simulink model "SF007A_SysFricLrng"  (R2013b)
settings: Solver=FixedStepDiscrete  SolverMode=SingleTasking  StartTime=0.0  StopTime=1  FixedStep=0.002  RelTol=1e-3
PostLoadFcn:
  | , if any(exist('dsrtsu_mdlpostloadfcn', 'file') == [2, 3, 6]), try dsrtsu_mdlpostloadfcn('Execute', bdroot); catch fprintf('Error in PostLoadFcn (dsrtsu_mdlpostloadfcn) for model "%s":\n %s\n', bdroot, lasterr); end, end,
values from neighbouring files (symbols this model uses):
  ARCHGLBPRM_100MILLISEC_SEC_F32 = DataDict.Constant    [SF007A_SysFricLrng_DataDict.m]
  ARCHGLBPRM_10MILLISEC_SEC_F32 = DataDict.Constant    [SF007A_SysFricLrng_DataDict.m]
  ARCHGLBPRM_180OVERPI_ULS_F32 = DataDict.Constant    [SF007A_SysFricLrng_DataDict.m]
  CONV100MICROSECTOSEC_ULS_F32 = DataDict.Constant    [SF007A_SysFricLrng_DataDict.m]
  FLTINJ_SYSFRICLRNG_SYSFRICOFFS = DataDict.Constant    [SF007A_SysFricLrng_DataDict.m]
  FricLrngData = DataDict.NVM    [SF007A_SysFricLrng_DataDict.m]
  HWPTNUM_CNT_U08 = DataDict.Constant    [SF007A_SysFricLrng_DataDict.m]
  HWPTNUMSUB1_CNT_U08 = DataDict.Constant    [SF007A_SysFricLrng_DataDict.m]
  HWVELDECDIR_ULS_U08 = DataDict.Constant    [SF007A_SysFricLrng_DataDict.m]
  HWVELINCDIR_ULS_U08 = DataDict.Constant    [SF007A_SysFricLrng_DataDict.m]
  IDXCALCNSCAGFAC_ULS_U08 = DataDict.Constant    [SF007A_SysFricLrng_DataDict.m]
  IDXSELN1_ULS_U08 = DataDict.Constant    [SF007A_SysFricLrng_DataDict.m]
  IDXSELN2_ULS_U08 = DataDict.Constant    [SF007A_SysFricLrng_DataDict.m]
  IDXSELN3_ULS_U08 = DataDict.Constant    [SF007A_SysFricLrng_DataDict.m]
  LRNGENASCAFAC_MILLISEC_U32 = DataDict.Constant    [SF007A_SysFricLrng_DataDict.m]
  SCAGFACQUARTER_CNT_F32 = DataDict.Constant    [SF007A_SysFricLrng_DataDict.m]
  SCAGFACTEN_CNT_U16 = DataDict.Constant    [SF007A_SysFricLrng_DataDict.m]
  SCAGFACVEHLATA_MTRPERSECSQD_F32 = DataDict.Constant    [SF007A_SysFricLrng_DataDict.m]
  SECIDXSELN_ULS_U08 = DataDict.Constant    [SF007A_SysFricLrng_DataDict.m]
  SysFricLrngBasLineEolFric = DataDict.Calibration    [SF007A_SysFricLrng_DataDict.m]
  SysFricLrngBasLineFric = DataDict.Calibration    [SF007A_SysFricLrng_DataDict.m]
  SysFricLrngBasLineHys = DataDict.Calibration    [SF007A_SysFricLrng_DataDict.m]
  SysFricLrngBasLineRngCntr = DataDict.Calibration    [SF007A_SysFricLrng_DataDict.m]
  SysFricLrngEolFricDifScagFac = DataDict.Calibration    [SF007A_SysFricLrng_DataDict.m]
  SysFricLrngFricChgWght = DataDict.Calibration    [SF007A_SysFricLrng_DataDict.m]
  SysFricLrngFricDiagcThd = DataDict.Calibration    [SF007A_SysFricLrng_DataDict.m]
  SysFricLrngFricDiagcTiThd = DataDict.Calibration    [SF007A_SysFricLrng_DataDict.m]
  SysFricLrngFricHysHwAgPt = DataDict.Calibration    [SF007A_SysFricLrng_DataDict.m]
  SysFricLrngGain = DataDict.Calibration    [SF007A_SysFricLrng_DataDict.m]
  SysFricLrngHwPosnAuthyThd = DataDict.Calibration    [SF007A_SysFricLrng_DataDict.m]
  SysFricLrngHwVelConstrLim = DataDict.Calibration    [SF007A_SysFricLrng_DataDict.m]
  SysFricLrngHwVelHiLim = DataDict.Calibration    [SF007A_SysFricLrng_DataDict.m]
  SysFricLrngHwVelLoLim = DataDict.Calibration    [SF007A_SysFricLrng_DataDict.m]
  SysFricLrngIgnCycFricChgLim = DataDict.Calibration    [SF007A_SysFricLrng_DataDict.m]
  SysFricLrngLatAHiLim = DataDict.Calibration    [SF007A_SysFricLrng_DataDict.m]
  SysFricLrngLatALoLim = DataDict.Calibration    [SF007A_SysFricLrng_DataDict.m]
  SysFricLrngMaskVehSpd = DataDict.Calibration    [SF007A_SysFricLrng_DataDict.m]
  SysFricLrngRngCntrThd = DataDict.Calibration    [SF007A_SysFricLrng_DataDict.m]
  SysFricLrngThd = DataDict.Calibration    [SF007A_SysFricLrng_DataDict.m]
  SysFricLrngTHiLim = DataDict.Calibration    [SF007A_SysFricLrng_DataDict.m]
  SysFricLrngTLoLim = DataDict.Calibration    [SF007A_SysFricLrng_DataDict.m]
  SysFricLrngVehSpd = DataDict.Calibration    [SF007A_SysFricLrng_DataDict.m]
  SYSFRICOFFSLIM_HWNWTMTR_F32 = DataDict.Constant    [SF007A_SysFricLrng_DataDict.m]
  VEHSPDPTNUM1_ULS_U08 = DataDict.Constant    [SF007A_SysFricLrng_DataDict.m]
  VEHSPDPTNUM2_ULS_U08 = DataDict.Constant    [SF007A_SysFricLrng_DataDict.m]
undefined symbols (not defined in the file or in its folder): NtcNr1, NtcSts1, SysFricLrngOperMod1
libraries: Fil x19, simulink x17, NxtrLim x10, NxtrAbslt x3, NxtrNvM x2, FixdToFloat x2, FloatToFixd x1, LnrIntrpn x1
(part 1 of 7)
settings Model: DSRTSU_INTERNAL_RTI_VER=370  DSRTSU_INTERNAL_RTI_TYPE=rti1401  Creator=fzv52m  LastModifiedBy=VZBTJX
settings Model: ModifiedHistory=|
  | Ver 004 Removed ignition latching of Friction Detection NTC to match software.
  | Limiting of P steps to one per ignition is being done with latching NTC allowing for the change
settings SolverCC: AutoInsertRateTranBlk=on  InsertRTBMode=Always
settings DataIOCC: LimitDataPoints=off  SaveFormat=Structure  ReturnWorkspaceOutputs=on
settings OptimizationCC: BlockReduction=off  InlineParams=on  ZeroExternalMemoryAtStartup=off  ZeroInternalMemoryAtStartup=off  OptimizeModelRefInitCode=on  LifeSpan=1
settings DebuggingCC: SignalInfNanChecking=error  SignalRangeChecking=warning  UnderspecifiedInitializationDetection=Simplified  SolverPrmCheckMsg=error  InheritedTsInSrcMsg=error  DiscreteInheritContinuousMsg=error  SingleTaskRateTransMsg=error  TasksWithSamePriorityMsg=error  SigSpecEnsureSampleTimeMsg=error  CheckMatrixSingularityMsg=error  ParameterUnderflowMsg=error  ParameterPrecisionLossMsg=error  ParameterTunabilityLossMsg=error  FixptConstUnderflowMsg=warning  FixptConstOverflowMsg=warning  VectorMatrixConversionMsg=error  SignalLabelMismatchMsg=error  UnconnectedInputMsg=error  UnconnectedOutputMsg=error  UnconnectedLineMsg=error  SFcnCompatibilityMsg=error  UniqueDataStoreMsg=warning  BusObjectLabelMismatch=error  RootOutportRequireBusObject=error  AssertControl=DisableAll  ModelReferenceIOMsg=error  ModelReferenceVersionMismatchMessage=warning  ModelReferenceIOMismatchMessage=error  ModelReferenceCSMismatchMessage=warning  ModelReferenceDataLoggingMessage=error  StateNameClashWarn=warning  StrictBusMsg=ErrorOnBusTreatedAsVector  NonBusSignalsTreatedAsBus=error  SFUnexpectedBacktrackingDiag=error  SFInvalidInputDataAccessInChartInitDiag=error  SFNoUnconditionalDefaultTransitionDiag=error  SFTransitionOutsideNaturalParentDiag=error  SFUnconditionalTransitionShadowingDiag=error  SFUndirectedBroadcastEventsDiag=error
settings ModelReferenceCC: ModelReferenceNumInstancesAllowed=Single
settings SFSimCC: SimGenImportedTypeDefs=on
settings RTWCC: SystemTargetFile=autosar.tlc  GenCodeOnly=on  TemplateMakefile=ert_default_tmf  Description=AUTOSAR  GenerateReport=on  ProcessScript=autosar_make_rtw_hook  LaunchReport=on
settings CodeAppCC: GenerateComments=off  IgnoreCustomStorageClasses=off  CustomSymbolStrType=$N$R$M  CustomSymbolStrBlkIO=$N$M  SimulinkBlockComments=off
settings STFCustomTargetCC: ParMdlRefBuildCompliant=on  CompOptLevelCompliant=on  IncludeMdlTerminateFcn=off  CombineOutputUpdateFcns=on  SuppressErrorStatus=on  ERTFirstTimeCompliant=on  ERTCustomFileBanners=on  SupportNonFinite=off  SupportComplex=off  SupportContinuousTime=off  SupportNonInlinedSFcns=off  MATLABClassNameForMDSCustomization=Simulink.SoftwareTarget.ERTCustomization  AutosarCompliant=on  GRTInterface=off  SystemTargetFile=autosar.tlc
settings ERTTargetCC: CodeReplacementLibrary=ANSI_C  ConcurrentExecutionCompliant=off  IncludeMdlTerminateFcn=off  SuppressErrorStatus=on  SupportNonFinite=off  SupportComplex=off  ModelStepFunctionPrototypeControlCompliant=off  CPPClassGenCompliant=off  AutosarCompliant=on  InlinedParameterPlacement=NonHierarchical  ERTCustomFileTemplate=example_file_process.tlc  EnableUserReplacementTypes=on

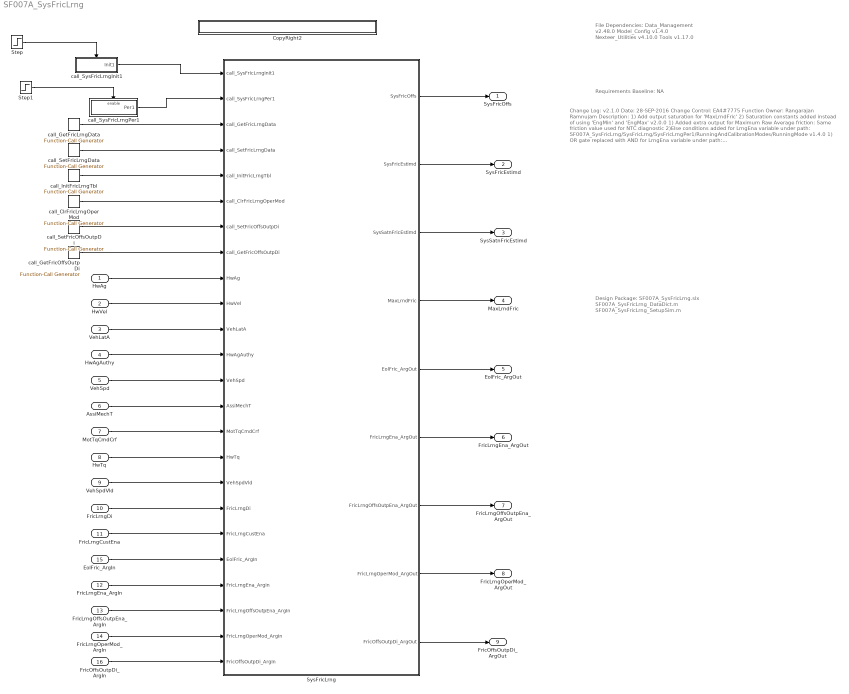
== system SF007A_SysFricLrng ==
  note: Requirements Baseline: NA
  note: File Dependencies:
      |
      | Data_Management v2.48.0
      | Model_Config v1.4.0
      | Nexteer_Utilities v4.10.0
      | Tools v1.17.0
  note: Change Log:
      |
      | v2.1.0
      | Date: 28-SEP-2016
      | Change Control: EA4#7775
      | Function Owner:  Rangarajan Ramnujam
      | Description:
      | 1) Add output saturation for 'MaxLrndFric'
      | 2) Saturation constants added instead of using 'EngMin' and 'EngMax'
      |
      | v2.0.0
      | 1) Added extra output for Maximum Raw Average friction: Same friction value used for NTC diagnostic
      | 2)Else conditions added for LrngEna variable under path:
      | SF007A_SysFricLrng/SysFricLrng/SysFricLrngPer1/RunningAndCalibrationModes/RunningMode
      |
      | v1.4.0
      | 1) OR gate replaced with AND for LrngEna variable under path:
      | SF007A_SysFricLrng/SysFricLrng/SysFricLrngPer1/RunningAndCalibrationModes
      | 2) Logic updated under path
      | SF007A_SysFricLrng/SysFricLrng/SysFricLrngPer1/RunningAndCalibrationModes/Running Mode
      | 3) Eng min to -127 and Eng max to 254 updated for PIM 'FilAvrgFric' in Data Dict
      | 4) Logic for Indices calculation updated under below path. This change needed only in model as
      |     model uses one based Index logic. No code change required for this.
      |     SF007A_SysFricLrng/SysFricLrng/SysFricLrngPer1/RunningAndCalibrationModes/FricLearning/Indices Calculation
      | - Changes are highlighted in red. Code change needed for above mentioned changes 1, 2, and 4.
      |
      | v1.3.1
      | Date: 18-JULY-2016
      | Change Control: EA4#6450
      | DRW:  Hari Prasad(KPIT)
      | Description:
      | - Anomaly EA4#6361 Fixing for Gate variable look up table indexing.
      |   Removed 'Gate_Cnt_T_u08' temporary data store memory block.
      |   Logic related to it has been updated.
      | - Changes are highlighted in red. No code change needed.
      |
      | v1.3.0
      | Date: 07-APR-2016
      | Change Control #4835:
      | DRW:  Muragesh Asundi
      | Description:
      | - List of issues fixed are available under
      |   Doc/SF007_FDD_Issues.xlsx/Issues in V1.2.0
      | - In below path, Changed Gate from PIM to port inside subsystem
      |  as PIM wholds extra increment inside while loop
      |   SF007A_SysFricLrng/SysFricLrng/SysFricLrngPer1/RunningAndCalibrationModes/
      |   FricLearning/Range Counter Manager/Range Counter Control
      |
      | v1.2.0
      | Date: 30-Mar-2016
      | Change Control #4835:
      | DR W:  Muragesh Asundi
      | Description:
      | - List of issues fixed are available under
      |   Doc/SF007_FDD_Issues.xlsx/Issues in V1.1.0
      | - 'SetFricLrngOperMod' renamed to 'SetFricLrngData'
      | - 'SetEolFric' removed and merged with 'SetFricLrngData'
      | - Following PIMs have been removed from model and DD
      | 'HwAgPrev', 'HwVelPrev', 'ColTq'
      | - Monotony of callibration table 'SysFricLrngFricHysHwAgPt'
      | changed to 'Strictly_Increasing'
      | - Init value of PIM 'TotCntr' changed to 1
      |
      | v1.1.0
      | Date: 25-Mar-2016
      | Change Control #4835:
      | DRW:  Hari Prasad
      | Description:
      | - List of issues fixed are available under
      |   Doc/SF007_FDD_Issues.xlsx
      | - Changes are highlighed in red color
      |
      | v1.0.0
      | Date: 11-Mar-2016
      | Change Control #2719:
      | DRW:  Hari Prasad, Muragesh Asundi
      | Description:
      | - Initial Release of EA4 from EA3 V008
  note: Design Package:
      |
      | SF007A_SysFricLrng.slx
      | SF007A_SysFricLrng_DataDict.m
      | SF007A_SysFricLrng_SetupSim.m
  HwAg : Inport
  HwVel : Inport  Port=2
  VehLatA : Inport  Port=3
  HwAgAuthy : Inport  Port=4
  VehSpd : Inport  Port=5
  AssiMechT : Inport  Port=6
  MotTqCmdCrf : Inport  Port=7
  HwTq : Inport  Port=8
  VehSpdVld : Inport  Port=9
  FricLrngDi : Inport  Port=10
  FricLrngCustEna : Inport  Port=11
  FricLrngEna_ArgIn : Inport  Port=12
  FricLrngOffsOutpEna_ArgIn : Inport  Port=13
  FricLrngOperMod_ArgIn : Inport  Port=14
  EolFric_ArgIn : Inport  Port=15
  FricOffsOutpDi_ArgIn : Inport  Port=16
  CopyRight2 : Subsystem  Description=|  mask(Copyright Information){none=on}
      | Copyright info block.                                               
      |                                                                     
      | Place copyright information at the top of every subsystem in design.
      mask prompts: none "No parameters"
      mask help: Place copyright information at the top of every subsystem in design.
      mask Display:
      | NxtrConf = 'Nexteer Confidential';
      | 
      | sys = bdroot; %handle for the current model ("system")
      | first = get_param(sys,'Created');
      | first = first(end-3:end);  %year is last four digits
      | 
      | last = get_param(sys,'LastModifiedDate');
      | if isempty(last)
      |     last = datestr(now,'yyyy');
      | else
      |     last = last(end-3:end);
      | end
      | 
      | if strcmp(first,last)
      |     fprintf('%s -- Copyright %s Nexteer',NxtrConf,first)
      | else
      |     fprintf('%s -- %s%s- %s Nexteer',NxtrConf,char(169),first,last)
      | end
  Step : Step  Time=.001  Before=1  After=0  SampleTime=0
  Step1 : Step  Time=.001  SampleTime=0
  SysFricLrng : Subsystem
  call_ClrFricLrngOperMod : simulink/Ports & Subsystems/Function-Call Generator  sample_time=0.010  numberOfIterations=1
  call_GetFricLrngData : simulink/Ports & Subsystems/Function-Call Generator  sample_time=0.010  numberOfIterations=1
  call_GetFricOffsOutpDi : simulink/Ports & Subsystems/Function-Call Generator  sample_time=0.010  numberOfIterations=1
  call_InitFricLrngTbl : simulink/Ports & Subsystems/Function-Call Generator  sample_time=0.010  numberOfIterations=1
  call_SetFricLrngData : simulink/Ports & Subsystems/Function-Call Generator  sample_time=0.010  numberOfIterations=1
  call_SetFricOffsOutpDi : simulink/Ports & Subsystems/Function-Call Generator  sample_time=0.010  numberOfIterations=1
  call_SysFricLrngInit1 : Subsystem  TreatAsAtomicUnit=on
  call_SysFricLrngPer1 : Subsystem  TreatAsAtomicUnit=on
  SysFricOffs : Outport
  SysFricEstimd : Outport  Port=2
  SysSatnFricEstimd : Outport  Port=3
  MaxLrndFric : Outport  Port=4
  EolFric_ArgOut : Outport  Port=5
  FricLrngEna_ArgOut : Outport  Port=6
  FricLrngOffsOutpEna_ArgOut : Outport  Port=7
  FricLrngOperMod_ArgOut : Outport  Port=8
  FricOffsOutpDi_ArgOut : Outport  Port=9
  wires:
  MotTqCmdCrf/1 -> SysFricLrng/15(MotTqCmdCrf)
  FricLrngDi/1 -> SysFricLrng/18(FricLrngDi)
  HwVel/1 -> SysFricLrng/10(HwVel)
  HwAg/1 -> SysFricLrng/9(HwAg)
  HwTq/1 -> SysFricLrng/16(HwTq)
  VehSpdVld/1 -> SysFricLrng/17(VehSpdVld)
  call_GetFricLrngData/1 -> SysFricLrng/3(call_GetFricLrngData)
  HwAgAuthy/1 -> SysFricLrng/12(HwAgAuthy)
  AssiMechT/1 -> SysFricLrng/14(AssiMechT)
  VehLatA/1 -> SysFricLrng/11(VehLatA)
  VehSpd/1 -> SysFricLrng/13(VehSpd)
  SysFricLrng/1(SysFricOffs) -> SysFricOffs/1
  SysFricLrng/3(SysSatnFricEstimd) -> SysSatnFricEstimd/1
  SysFricLrng/2(SysFricEstimd) -> SysFricEstimd/1
  FricLrngCustEna/1 -> SysFricLrng/19(FricLrngCustEna)
  call_SetFricLrngData/1 -> SysFricLrng/4(call_SetFricLrngData)
  call_InitFricLrngTbl/1 -> SysFricLrng/5(call_InitFricLrngTbl)
  call_SetFricOffsOutpDi/1 -> SysFricLrng/7(call_SetFricOffsOutpDi)
  call_GetFricOffsOutpDi/1 -> SysFricLrng/8(call_GetFricOffsOutpDi)
  call_ClrFricLrngOperMod/1 -> SysFricLrng/6(call_ClrFricLrngOperMod)
  SysFricLrng/6(FricLrngEna_ArgOut) -> FricLrngEna_ArgOut/1
  SysFricLrng/8(FricLrngOperMod_ArgOut) -> FricLrngOperMod_ArgOut/1
  SysFricLrng/7(FricLrngOffsOutpEna_ArgOut) -> FricLrngOffsOutpEna_ArgOut/1
  SysFricLrng/9(FricOffsOutpDi_ArgOut) -> FricOffsOutpDi_ArgOut/1
  SysFricLrng/5(EolFric_ArgOut) -> EolFric_ArgOut/1
  FricLrngEna_ArgIn/1 -> SysFricLrng/21(FricLrngEna_ArgIn)
  FricLrngOffsOutpEna_ArgIn/1 -> SysFricLrng/22(FricLrngOffsOutpEna_ArgIn)
  FricLrngOperMod_ArgIn/1 -> SysFricLrng/23(FricLrngOperMod_ArgIn)
  EolFric_ArgIn/1 -> SysFricLrng/20(EolFric_ArgIn)
  FricOffsOutpDi_ArgIn/1 -> SysFricLrng/24(FricOffsOutpDi_ArgIn)
  call_SysFricLrngInit1/1(Init1) -> SysFricLrng/1(call_SysFricLrngInit1)
  Step/1 -> call_SysFricLrngInit1/Enable
  call_SysFricLrngPer1/1(Per1) -> SysFricLrng/2(call_SysFricLrngPer1)
  Step1/1 -> call_SysFricLrngPer1/Enable
  SysFricLrng/4(MaxLrndFric) -> MaxLrndFric/1

== system SF007A_SysFricLrng/CopyRight2 ==

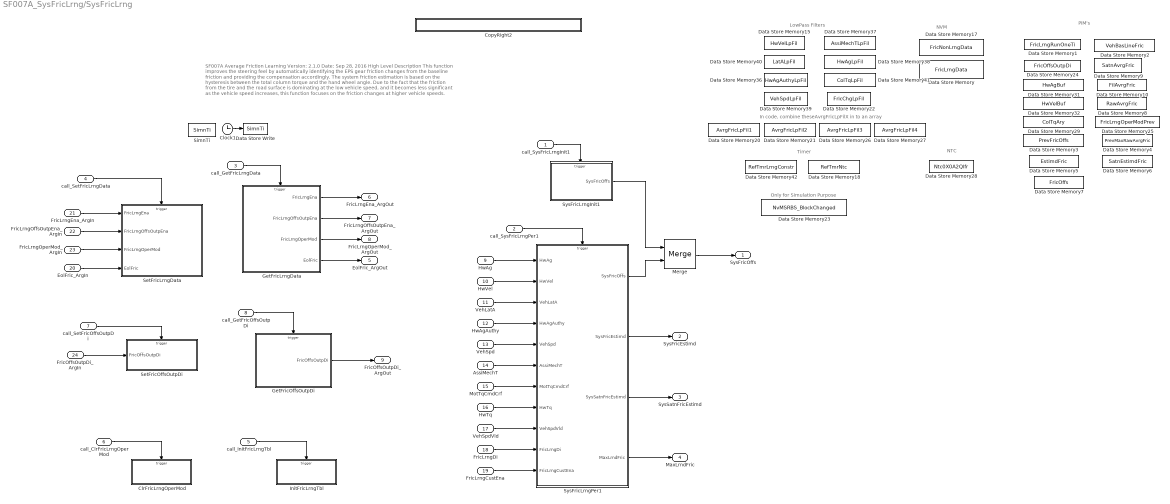
== system SF007A_SysFricLrng/SysFricLrng ==
  note: In code, combine theseAvrgFricLpFilX in to an array
  note: Only for Simulation Purpose
  note: PIM's
  note: Timer
  note: LowPass Filters
  note: NVM
  note: SF007A  Average Friction Learning
      | Version: 2.1.0          																															 					Date: Sep 28,  2016
      |
      | High Level Description
      |
      | This function improves the steering feel by automatically identifying the EPS gear friction changes from the baseline friction and providing the compensation accordingly. The system friction estimation
      |  is based on the hysteresis between the total column torque and the hand wheel angle. Due to the fact that the friction from the tire and the road surface is dominating at the low vehicle speed,  and it
      | becomes less significant as the vehicle speed increases, this function focuses on the friction changes at higher vehicle speeds.
  note: NTC
  call_SysFricLrngInit1 : Inport
  call_SysFricLrngPer1 : Inport  Port=2
  call_GetFricLrngData : Inport  Port=3
  call_SetFricLrngData : Inport  Port=4
  call_InitFricLrngTbl : Inport  Port=5
  call_ClrFricLrngOperMod : Inport  Port=6
  call_SetFricOffsOutpDi : Inport  Port=7
  call_GetFricOffsOutpDi : Inport  Port=8
  HwAg : Inport  Port=9
  HwVel : Inport  Port=10
  VehLatA : Inport  Port=11
  HwAgAuthy : Inport  Port=12
  VehSpd : Inport  Port=13
  AssiMechT : Inport  Port=14
  MotTqCmdCrf : Inport  Port=15
  HwTq : Inport  Port=16
  VehSpdVld : Inport  Port=17
  FricLrngDi : Inport  Port=18
  FricLrngCustEna : Inport  Port=19
  EolFric_ArgIn : Inport  Port=20
  FricLrngEna_ArgIn : Inport  Port=21
  FricLrngOffsOutpEna_ArgIn : Inport  Port=22
  FricLrngOperMod_ArgIn : Inport  Port=23
  FricOffsOutpDi_ArgIn : Inport  Port=24
  Clock1 : Clock
  ClrFricLrngOperMod : Subsystem
  CopyRight2 : Subsystem  Description=|  mask(Copyright Information){none=on}
      | Copyright info block.                                               
      |                                                                     
      | Place copyright information at the top of every subsystem in design.
      mask prompts: none "No parameters"
      mask help: Place copyright information at the top of every subsystem in design.
      mask Display:
      | NxtrConf = 'Nexteer Confidential';
      | 
      | sys = bdroot; %handle for the current model ("system")
      | first = get_param(sys,'Created');
      | if(isempty(first))
      |     first = datestr(now,'yyyy');
      | else
      |     first = first(end-3:end);  %year is last four digits
      | end
      | 
      | last = get_param(sys,'LastModifiedDate');
      | if isempty(last)
      |     last = datestr(now,'yyyy');
      | else
      |     last = last(end-3:end);
      | end
      | 
      | if strcmp(first,last)
      |     fprintf('%s -- Copyright %s Nexteer',NxtrConf,first)
      | else
      |     fprintf('%s -- %s%s- %s Nexteer',NxtrConf,char(169),first,last)
      | end
  Data Store Memory : DataStoreMemory  DataStoreName=FricLrngData  InitialValue=[]  OutDataTypeStr=Bus: SysFricDataRec1  StateMustResolveToSignalObject=on
  Data Store Memory1 : DataStoreMemory  DataStoreName=FricLrngRunOneTi  StateMustResolveToSignalObject=on
  Data Store Memory10 : DataStoreMemory  DataStoreName=FilAvrgFric  InitialValue=[0 0 0 0]  OutDataTypeStr=single  StateMustResolveToSignalObject=on
  Data Store Memory15 : DataStoreMemory  DataStoreName=HwVelLpFil  InitialValue=struct('FilSt',single(0),'FilGain',single(0))  OutDataTypeStr=Bus: FilLpRec1  StateMustResolveToSignalObject=on
  Data Store Memory17 : DataStoreMemory  DataStoreName=FricNonLrngData  InitialValue=[]  OutDataTypeStr=Bus: SysFricNonLrngDataRec1  StateMustResolveToSignalObject=on
  Data Store Memory18 : DataStoreMemory  DataStoreName=RefTmrNtc  StateMustResolveToSignalObject=on
  Data Store Memory2 : DataStoreMemory  DataStoreName=VehBasLineFric  InitialValue=[0 0 0 0]  StateMustResolveToSignalObject=on
  Data Store Memory20 : DataStoreMemory  DataStoreName=AvrgFricLpFil1  InitialValue=struct('FilSt',single(0),'FilGain',single(0))  OutDataTypeStr=Bus: FilLpRec1  StateMustResolveToSignalObject=on
  Data Store Memory21 : DataStoreMemory  DataStoreName=AvrgFricLpFil2  InitialValue=struct('FilSt',single(0),'FilGain',single(0))  OutDataTypeStr=Bus: FilLpRec1  StateMustResolveToSignalObject=on
  Data Store Memory22 : DataStoreMemory  DataStoreName=FricChgLpFil  InitialValue=struct('FilSt',single(0),'FilGain',single(0))  OutDataTypeStr=Bus: FilLpRec1  StateMustResolveToSignalObject=on
  Data Store Memory23 : DataStoreMemory  DataStoreName=NvMSRBS_BlockChanged
  Data Store Memory24 : DataStoreMemory  DataStoreName=FricOffsOutpDi  StateMustResolveToSignalObject=on
  Data Store Memory25 : DataStoreMemory  DataStoreName=FricLrngOperModPrev  InitialValue=[]  StateMustResolveToSignalObject=on
  Data Store Memory26 : DataStoreMemory  DataStoreName=AvrgFricLpFil3  InitialValue=struct('FilSt',single(0),'FilGain',single(0))  OutDataTypeStr=Bus: FilLpRec1  StateMustResolveToSignalObject=on
  Data Store Memory27 : DataStoreMemory  DataStoreName=AvrgFricLpFil4  InitialValue=struct('FilSt',single(0),'FilGain',single(0))  OutDataTypeStr=Bus: FilLpRec1  StateMustResolveToSignalObject=on
  Data Store Memory28 : DataStoreMemory  DataStoreName=Ntc0X0A2Qlfr  InitialValue=SigQlfr1.SIGQLFR_NORES
  Data Store Memory29 : DataStoreMemory  DataStoreName=ColTqAry  InitialValue=[]  StateMustResolveToSignalObject=on
  Data Store Memory3 : DataStoreMemory  DataStoreName=PrevFricOffs  InitialValue=[]  StateMustResolveToSignalObject=on
  Data Store Memory31 : DataStoreMemory  DataStoreName=HwAgBuf  InitialValue=[0 0 0 0 0 0 0 0 0 0 0 0]  StateMustResolveToSignalObject=on
  Data Store Memory32 : DataStoreMemory  DataStoreName=HwVelBuf  InitialValue=[0 0 0 0 0 0 0 0 0 0 0 0]  StateMustResolveToSignalObject=on
  Data Store Memory36 : DataStoreMemory  DataStoreName=HwAgAuthyLpFil  InitialValue=struct('FilSt',single(0),'FilGain',single(0))  OutDataTypeStr=Bus: FilLpRec1  StateMustResolveToSignalObject=on
  Data Store Memory37 : DataStoreMemory  DataStoreName=AssiMechTLpFil  InitialValue=struct('FilSt',single(0),'FilGain',single(0))  OutDataTypeStr=Bus: FilLpRec1  StateMustResolveToSignalObject=on
  Data Store Memory38 : DataStoreMemory  DataStoreName=HwAgLpFil  InitialValue=struct('FilSt',single(0),'FilGain',single(0))  OutDataTypeStr=Bus: FilLpRec1  StateMustResolveToSignalObject=on
  Data Store Memory39 : DataStoreMemory  DataStoreName=VehSpdLpFil  InitialValue=struct('FilSt',single(0),'FilGain',single(0))  OutDataTypeStr=Bus: FilLpRec1  StateMustResolveToSignalObject=on
  Data Store Memory4 : DataStoreMemory  DataStoreName=PrevMaxRawAvrgFric  InitialValue=[]  OutDataTypeStr=single  StateMustResolveToSignalObject=on
  Data Store Memory40 : DataStoreMemory  DataStoreName=LatALpFil  InitialValue=struct('FilSt',single(0),'FilGain',single(0))  OutDataTypeStr=Bus: FilLpRec1  StateMustResolveToSignalObject=on
  Data Store Memory41 : DataStoreMemory  DataStoreName=ColTqLpFil  InitialValue=struct('FilSt',single(0),'FilGain',single(0))  OutDataTypeStr=Bus: FilLpRec1  StateMustResolveToSignalObject=on
  Data Store Memory42 : DataStoreMemory  DataStoreName=RefTmrLrngConstr  StateMustResolveToSignalObject=on
  Data Store Memory5 : DataStoreMemory  DataStoreName=EstimdFric  InitialValue=[]  OutDataTypeStr=single  StateMustResolveToSignalObject=on
  Data Store Memory6 : DataStoreMemory  DataStoreName=SatnEstimdFric  InitialValue=[]  OutDataTypeStr=single  StateMustResolveToSignalObject=on
  Data Store Memory7 : DataStoreMemory  DataStoreName=FricOffs  InitialValue=[]  OutDataTypeStr=single  StateMustResolveToSignalObject=on
  Data Store Memory8 : DataStoreMemory  DataStoreName=RawAvrgFric  InitialValue=[0 0 0 0]  OutDataTypeStr=single  StateMustResolveToSignalObject=on
  Data Store Memory9 : DataStoreMemory  DataStoreName=SatnAvrgFric  InitialValue=[0 0 0 0]  StateMustResolveToSignalObject=on
  Data Store Write : DataStoreWrite  DataStoreName=SimnTi
  GetFricLrngData : Subsystem
  GetFricOffsOutpDi : Subsystem
  InitFricLrngTbl : Subsystem
  Merge : Merge
  SetFricLrngData : Subsystem
  SetFricOffsOutpDi : Subsystem
  SimnTi : DataStoreMemory  DataStoreName=SimnTi
  SysFricLrngInit1 : Subsystem
  SysFricLrngPer1 : Subsystem
  SysFricOffs : Outport
  SysFricEstimd : Outport  Port=2
  SysSatnFricEstimd : Outport  Port=3
  MaxLrndFric : Outport  Port=4
  EolFric_ArgOut : Outport  Port=5
  FricLrngEna_ArgOut : Outport  Port=6
  FricLrngOffsOutpEna_ArgOut : Outport  Port=7
  FricLrngOperMod_ArgOut : Outport  Port=8
  FricOffsOutpDi_ArgOut : Outport  Port=9
  wires:
  call_SysFricLrngInit1/1 -> SysFricLrngInit1/Trigger
  HwAg/1 -> SysFricLrngPer1/1(HwAg)
  HwVel/1 -> SysFricLrngPer1/2(HwVel)
  VehLatA/1 -> SysFricLrngPer1/3(VehLatA)
  HwAgAuthy/1 -> SysFricLrngPer1/4(HwAgAuthy)
  VehSpd/1 -> SysFricLrngPer1/5(VehSpd)
  AssiMechT/1 -> SysFricLrngPer1/6(AssiMechT)
  MotTqCmdCrf/1 -> SysFricLrngPer1/7(MotTqCmdCrf)
  HwTq/1 -> SysFricLrngPer1/8(HwTq)
  VehSpdVld/1 -> SysFricLrngPer1/9(VehSpdVld)
  FricLrngDi/1 -> SysFricLrngPer1/10(FricLrngDi)
  call_SysFricLrngPer1/1 -> SysFricLrngPer1/Trigger
  Clock1/1 -> Data Store Write/1
  SysFricLrngPer1/3(SysSatnFricEstimd) -> SysSatnFricEstimd/1
  SysFricLrngPer1/2(SysFricEstimd) -> SysFricEstimd/1
  FricLrngCustEna/1 -> SysFricLrngPer1/11(FricLrngCustEna)
  call_SetFricLrngData/1 -> SetFricLrngData/Trigger
  call_GetFricLrngData/1 -> GetFricLrngData/Trigger
  call_SetFricOffsOutpDi/1 -> SetFricOffsOutpDi/Trigger
  call_GetFricOffsOutpDi/1 -> GetFricOffsOutpDi/Trigger
  call_InitFricLrngTbl/1 -> InitFricLrngTbl/Trigger
  call_ClrFricLrngOperMod/1 -> ClrFricLrngOperMod/Trigger
  GetFricLrngData/1(FricLrngEna) -> FricLrngEna_ArgOut/1
  GetFricLrngData/3(FricLrngOperMod) -> FricLrngOperMod_ArgOut/1
  GetFricLrngData/2(FricLrngOffsOutpEna) -> FricLrngOffsOutpEna_ArgOut/1
  FricLrngEna_ArgIn/1 -> SetFricLrngData/1(FricLrngEna)
  FricLrngOperMod_ArgIn/1 -> SetFricLrngData/3(FricLrngOperMod)
  FricLrngOffsOutpEna_ArgIn/1 -> SetFricLrngData/2(FricLrngOffsOutpEna)
  FricOffsOutpDi_ArgIn/1 -> SetFricOffsOutpDi/1(FricOffsOutpDi)
  GetFricOffsOutpDi/1(FricOffsOutpDi) -> FricOffsOutpDi_ArgOut/1
  GetFricLrngData/4(EolFric) -> EolFric_ArgOut/1
  SysFricLrngInit1/1(SysFricOffs) -> Merge/1
  SysFricLrngPer1/1(SysFricOffs) -> Merge/2
  Merge/1 -> SysFricOffs/1
  EolFric_ArgIn/1 -> SetFricLrngData/4(EolFric)
  SysFricLrngPer1/4(MaxLrndFric) -> MaxLrndFric/1

== system SF007A_SysFricLrng/call_SysFricLrngInit1 ==
  Enable : EnablePort
  CopyRight2 : Subsystem  Description=|  mask(Copyright Information){none=on}
      | Copyright info block.                                               
      |                                                                     
      | Place copyright information at the top of every subsystem in design.
      mask prompts: none "No parameters"
      mask help: Place copyright information at the top of every subsystem in design.
      mask Display:
      | NxtrConf = 'Nexteer Confidential';
      | 
      | sys = bdroot; %handle for the current model ("system")
      | first = get_param(sys,'Created');
      | if(isempty(first))
      |     first = datestr(now,'yyyy');
      | else
      |     first = first(end-3:end);  %year is last four digits
      | end
      | 
      | last = get_param(sys,'LastModifiedDate');
      | if isempty(last)
      |     last = datestr(now,'yyyy');
      | else
      |     last = last(end-3:end);
      | end
      | 
      | if strcmp(first,last)
      |     fprintf('%s -- Copyright %s Nexteer',NxtrConf,first)
      | else
      |     fprintf('%s -- %s%s- %s Nexteer',NxtrConf,char(169),first,last)
      | end
  Function-Call Generator : simulink/Ports & Subsystems/Function-Call Generator  sample_time=.01  numberOfIterations=1
  Init1 : Outport
  wires:
  Function-Call Generator/1 -> Init1/1

== system SF007A_SysFricLrng/call_SysFricLrngPer1 ==
  Enable : EnablePort
  CopyRight2 : Subsystem  Description=|  mask(Copyright Information){none=on}
      | Copyright info block.                                               
      |                                                                     
      | Place copyright information at the top of every subsystem in design.
      mask prompts: none "No parameters"
      mask help: Place copyright information at the top of every subsystem in design.
      mask Display:
      | NxtrConf = 'Nexteer Confidential';
      | 
      | sys = bdroot; %handle for the current model ("system")
      | first = get_param(sys,'Created');
      | if(isempty(first))
      |     first = datestr(now,'yyyy');
      | else
      |     first = first(end-3:end);  %year is last four digits
      | end
      | 
      | last = get_param(sys,'LastModifiedDate');
      | if isempty(last)
      |     last = datestr(now,'yyyy');
      | else
      |     last = last(end-3:end);
      | end
      | 
      | if strcmp(first,last)
      |     fprintf('%s -- Copyright %s Nexteer',NxtrConf,first)
      | else
      |     fprintf('%s -- %s%s- %s Nexteer',NxtrConf,char(169),first,last)
      | end
  Function-Call Generator : simulink/Ports & Subsystems/Function-Call Generator  sample_time=.01  numberOfIterations=1
  Per1 : Outport
  wires:
  Function-Call Generator/1 -> Per1/1

== system SF007A_SysFricLrng/SysFricLrng/ClrFricLrngOperMod ==
  note: Set Ram Block Status for 'FricLrngData' moved to Init
  function : TriggerPort  TriggerType=function-call
  Constant1 : Constant  Value=false  OutDataTypeStr=boolean
      settings: AttributesFormatString=%<OutDataTypeStr>
  CopyRight2 : Subsystem  Description=|  mask(Copyright Information){none=on}
      | Copyright info block.                                               
      |                                                                     
      | Place copyright information at the top of every subsystem in design.
      mask prompts: none "No parameters"
      mask help: Place copyright information at the top of every subsystem in design.
      mask Display:
      | NxtrConf = 'Nexteer Confidential';
      | 
      | sys = bdroot; %handle for the current model ("system")
      | first = get_param(sys,'Created');
      | if(isempty(first))
      |     first = datestr(now,'yyyy');
      | else
      |     first = first(end-3:end);  %year is last four digits
      | end
      | 
      | last = get_param(sys,'LastModifiedDate');
      | if isempty(last)
      |     last = datestr(now,'yyyy');
      | else
      |     last = last(end-3:end);
      | end
      | 
      | if strcmp(first,last)
      |     fprintf('%s -- Copyright %s Nexteer',NxtrConf,first)
      | else
      |     fprintf('%s -- %s%s- %s Nexteer',NxtrConf,char(169),first,last)
      | end
  Data Store Read : DataStoreRead  DataStoreName=FricLrngData  DataStoreElements=FricLrngData.SysFricLrngOperMod
  Data Store Write : DataStoreWrite  DataStoreName=FricLrngOperModPrev
  Data Store Write1 : DataStoreWrite  DataStoreName=FricLrngData  DataStoreElements=FricLrngData.SysFricLrngOperMod
  Data Store Write2 : DataStoreWrite  DataStoreName=FricLrngRunOneTi
  Enumerated Constant : simulink/Sources/Enumerated Constant  OutDataTypeStr=Enum: SysFricLrngOperMod1  Value=SysFricLrngOperMod1.SYSFRICLRNGOPERMOD_CLEAR  SampleTime=inf
  wires:
  Constant1/1 -> Data Store Write2/1
  Enumerated Constant/1 -> Data Store Write1/1
  Data Store Read/1 -> Data Store Write/1

== system SF007A_SysFricLrng/SysFricLrng/CopyRight2 ==

== system SF007A_SysFricLrng/SysFricLrng/GetFricLrngData ==
  note: Get NVM Data
  function : TriggerPort  TriggerType=function-call
  CopyRight2 : Subsystem  Description=|  mask(Copyright Information){none=on}
      | Copyright info block.                                               
      |                                                                     
      | Place copyright information at the top of every subsystem in design.
      mask prompts: none "No parameters"
      mask help: Place copyright information at the top of every subsystem in design.
      mask Display:
      | NxtrConf = 'Nexteer Confidential';
      | 
      | sys = bdroot; %handle for the current model ("system")
      | first = get_param(sys,'Created');
      | first = first(end-3:end);  %year is last four digits
      | 
      | last = get_param(sys,'LastModifiedDate');
      | if isempty(last)
      |     last = datestr(now,'yyyy');
      | else
      |     last = last(end-3:end);
      | end
      | 
      | if strcmp(first,last)
      |     fprintf('%s -- Copyright %s Nexteer',NxtrConf,first)
      | else
      |     fprintf('%s -- %s%s- %s Nexteer',NxtrConf,char(169),first,last)
      | end
  Data Store Read : DataStoreRead  DataStoreName=FricLrngData  DataStoreElements=FricLrngData.SysFricLrngOperMod
  Data Store Read1 : DataStoreRead  DataStoreName=FricNonLrngData  DataStoreElements=FricNonLrngData.EnaFricLrng#FricNonLrngData.EnaFricOffsOutp#FricNonLrngData.EolFric
  FricLrngEna : Outport
  FricLrngOffsOutpEna : Outport  Port=2
  FricLrngOperMod : Outport  Port=3
  EolFric : Outport  Port=4
  wires:
  Data Store Read/1 -> FricLrngOperMod/1
  Data Store Read1/1 -> FricLrngEna/1
  Data Store Read1/2 -> FricLrngOffsOutpEna/1
  Data Store Read1/3 -> EolFric/1

== system SF007A_SysFricLrng/SysFricLrng/GetFricOffsOutpDi ==
  function : TriggerPort  TriggerType=function-call
  CopyRight2 : Subsystem  Description=|  mask(Copyright Information){none=on}
      | Copyright info block.                                               
      |                                                                     
      | Place copyright information at the top of every subsystem in design.
      mask prompts: none "No parameters"
      mask help: Place copyright information at the top of every subsystem in design.
      mask Display:
      | NxtrConf = 'Nexteer Confidential';
      | 
      | sys = bdroot; %handle for the current model ("system")
      | first = get_param(sys,'Created');
      | first = first(end-3:end);  %year is last four digits
      | 
      | last = get_param(sys,'LastModifiedDate');
      | if isempty(last)
      |     last = datestr(now,'yyyy');
      | else
      |     last = last(end-3:end);
      | end
      | 
      | if strcmp(first,last)
      |     fprintf('%s -- Copyright %s Nexteer',NxtrConf,first)
      | else
      |     fprintf('%s -- %s%s- %s Nexteer',NxtrConf,char(169),first,last)
      | end
  Data Store Read1 : DataStoreRead  DataStoreName=FricOffsOutpDi
  FricOffsOutpDi : Outport
  wires:
  Data Store Read1/1 -> FricOffsOutpDi/1

== system SF007A_SysFricLrng/SysFricLrng/InitFricLrngTbl ==
  note: Set Ram Block Status moved to Init
  function : TriggerPort  TriggerType=function-call
  Constant1 : Constant  Value=false  OutDataTypeStr=boolean
      settings: AttributesFormatString=%<OutDataTypeStr>
  CopyRight2 : Subsystem  Description=|  mask(Copyright Information){none=on}
      | Copyright info block.                                               
      |                                                                     
      | Place copyright information at the top of every subsystem in design.
      mask prompts: none "No parameters"
      mask help: Place copyright information at the top of every subsystem in design.
      mask Display:
      | NxtrConf = 'Nexteer Confidential';
      | 
      | sys = bdroot; %handle for the current model ("system")
      | first = get_param(sys,'Created');
      | if(isempty(first))
      |     first = datestr(now,'yyyy');
      | else
      |     first = first(end-3:end);  %year is last four digits
      | end
      | 
      | last = get_param(sys,'LastModifiedDate');
      | if isempty(last)
      |     last = datestr(now,'yyyy');
      | else
      |     last = last(end-3:end);
      | end
      | 
      | if strcmp(first,last)
      |     fprintf('%s -- Copyright %s Nexteer',NxtrConf,first)
      | else
      |     fprintf('%s -- %s%s- %s Nexteer',NxtrConf,char(169),first,last)
      | end
  Data Store Read : DataStoreRead  DataStoreName=FricLrngData  DataStoreElements=FricLrngData.SysFricLrngOperMod
  Data Store Write : DataStoreWrite  DataStoreName=FricLrngOperModPrev
  Data Store Write1 : DataStoreWrite  DataStoreName=FricLrngData  DataStoreElements=FricLrngData.SysFricLrngOperMod
  Data Store Write2 : DataStoreWrite  DataStoreName=FricLrngRunOneTi
  Enumerated Constant : simulink/Sources/Enumerated Constant  OutDataTypeStr=Enum: SysFricLrngOperMod1  Value=SysFricLrngOperMod1.SYSFRICLRNGOPERMOD_BASELINE  SampleTime=inf
  wires:
  Data Store Read/1 -> Data Store Write/1
  Enumerated Constant/1 -> Data Store Write1/1
  Constant1/1 -> Data Store Write2/1

== system SF007A_SysFricLrng/SysFricLrng/SetFricLrngData ==
  note: Set Ram Block Status for 'FricLrngData' moved to Init
  note: update NVM
  FricLrngEna : Inport
  FricLrngOffsOutpEna : Inport  Port=2
  FricLrngOperMod : Inport  Port=3
  EolFric : Inport  Port=4
  function : TriggerPort  TriggerType=function-call
  Constant1 : Constant  Value=true  OutDataTypeStr=boolean
      settings: AttributesFormatString=%<OutDataTypeStr>
  CopyRight2 : Subsystem  Description=|  mask(Copyright Information){none=on}
      | Copyright info block.                                               
      |                                                                     
      | Place copyright information at the top of every subsystem in design.
      mask prompts: none "No parameters"
      mask help: Place copyright information at the top of every subsystem in design.
      mask Display:
      | NxtrConf = 'Nexteer Confidential';
      | 
      | sys = bdroot; %handle for the current model ("system")
      | first = get_param(sys,'Created');
      | first = first(end-3:end);  %year is last four digits
      | 
      | last = get_param(sys,'LastModifiedDate');
      | if isempty(last)
      |     last = datestr(now,'yyyy');
      | else
      |     last = last(end-3:end);
      | end
      | 
      | if strcmp(first,last)
      |     fprintf('%s -- Copyright %s Nexteer',NxtrConf,first)
      | else
      |     fprintf('%s -- %s%s- %s Nexteer',NxtrConf,char(169),first,last)
      | end
  Data Store Write : DataStoreWrite  DataStoreName=FricLrngOperModPrev
  Data Store Write1 : DataStoreWrite  DataStoreName=FricLrngData  DataStoreElements=FricLrngData.SysFricLrngOperMod
  Data Store Write3 : DataStoreWrite  DataStoreName=FricNonLrngData  DataStoreElements=FricNonLrngData.EnaFricLrng#FricNonLrngData.EnaFricOffsOutp#FricNonLrngData.EolFric
  Set Ram Block Status1 : NxtrNvM/Set Ram Block Status  FuncName=Set Ram Block Status  NvMBlockName=FricNonLrngData  VoidFuncRtn=on  BlockChanged_DSN=NvMSRBS_BlockChanged  Return_DSN=NvMSRBS_Return
      settings: AttributesFormatString=%<FuncName>
  wires:
  Constant1/1 -> Set Ram Block Status1/1
  FricLrngOperMod/1 -> Data Store Write/1, Data Store Write1/1
  FricLrngEna/1 -> Data Store Write3/1
  FricLrngOffsOutpEna/1 -> Data Store Write3/2
  EolFric/1 -> Data Store Write3/3

== system SF007A_SysFricLrng/SysFricLrng/SetFricOffsOutpDi ==
  FricOffsOutpDi : Inport
  function : TriggerPort  TriggerType=function-call
  CopyRight2 : Subsystem  Description=|  mask(Copyright Information){none=on}
      | Copyright info block.                                               
      |                                                                     
      | Place copyright information at the top of every subsystem in design.
      mask prompts: none "No parameters"
      mask help: Place copyright information at the top of every subsystem in design.
      mask Display:
      | NxtrConf = 'Nexteer Confidential';
      | 
      | sys = bdroot; %handle for the current model ("system")
      | first = get_param(sys,'Created');
      | first = first(end-3:end);  %year is last four digits
      | 
      | last = get_param(sys,'LastModifiedDate');
      | if isempty(last)
      |     last = datestr(now,'yyyy');
      | else
      |     last = last(end-3:end);
      | end
      | 
      | if strcmp(first,last)
      |     fprintf('%s -- Copyright %s Nexteer',NxtrConf,first)
      | else
      |     fprintf('%s -- %s%s- %s Nexteer',NxtrConf,char(169),first,last)
      | end
  Data Store Write : DataStoreWrite  DataStoreName=FricOffsOutpDi
  wires:
  FricOffsOutpDi/1 -> Data Store Write/1

== system SF007A_SysFricLrng/SysFricLrng/SysFricLrngInit1 ==
  note: These 4 filters can be combined into array[4] of structures and initialization value be assigned from NVM varibale FricLrngData.VehLrndFric[] as part of 'Initialzation' for loop.
  function : TriggerPort  TriggerType=function-call
  AssiMechTLpFil : Fil/FilLpInit  Ic=0  Ts=ARCHGLBPRM_10MILLISEC_SEC_F32  Freq=SysFricLrngDataPrepLpFilFrq  StVar=AssiMechTLpFil
  AvrgFricLpFil1 : Fil/FilLpInit  Ic=0  Ts=ARCHGLBPRM_10MILLISEC_SEC_F32  Freq=SysFricLrngAvrgFricFrq  StVar=AvrgFricLpFil1
  AvrgFricLpFil2 : Fil/FilLpInit  Ic=0  Ts=ARCHGLBPRM_10MILLISEC_SEC_F32  Freq=SysFricLrngAvrgFricFrq  StVar=AvrgFricLpFil2
  AvrgFricLpFil3 : Fil/FilLpInit  Ic=0  Ts=ARCHGLBPRM_10MILLISEC_SEC_F32  Freq=SysFricLrngAvrgFricFrq  StVar=AvrgFricLpFil3
  AvrgFricLpFil4 : Fil/FilLpInit  Ic=0  Ts=ARCHGLBPRM_10MILLISEC_SEC_F32  Freq=SysFricLrngAvrgFricFrq  StVar=AvrgFricLpFil4
  ColTqLpFil : Fil/FilLpInit  Ic=0  Ts=ARCHGLBPRM_10MILLISEC_SEC_F32  Freq=SysFricLrngDataPrepLpFilFrq  StVar=ColTqLpFil
  Constant : Constant  Value=VEHSPDPTNUM1_ULS_U08
  Constant1 : Constant  Value=true  OutDataTypeStr=boolean
      settings: AttributesFormatString=%<OutDataTypeStr>
  CopyRight2 : Subsystem  Description=|  mask(Copyright Information){none=on}
      | Copyright info block.                                               
      |                                                                     
      | Place copyright information at the top of every subsystem in design.
      mask prompts: none "No parameters"
      mask help: Place copyright information at the top of every subsystem in design.
      mask Display:
      | NxtrConf = 'Nexteer Confidential';
      | 
      | sys = bdroot; %handle for the current model ("system")
      | first = get_param(sys,'Created');
      | if(isempty(first))
      |     first = datestr(now,'yyyy');
      | else
      |     first = first(end-3:end);  %year is last four digits
      | end
      | 
      | last = get_param(sys,'LastModifiedDate');
      | if isempty(last)
      |     last = datestr(now,'yyyy');
      | else
      |     last = last(end-3:end);
      | end
      | 
      | if strcmp(first,last)
      |     fprintf('%s -- Copyright %s Nexteer',NxtrConf,first)
      | else
      |     fprintf('%s -- %s%s- %s Nexteer',NxtrConf,char(169),first,last)
      | end
  Data Store Read : DataStoreRead  DataStoreName=FricLrngData  DataStoreElements=FricLrngData.SysFricLrngOperMod
  Data Store Read1 : DataStoreRead  DataStoreName=FricLrngData  DataStoreElements=FricLrngData.FricOffs
  Data Store Write : DataStoreWrite  DataStoreName=FricLrngOperModPrev
  Data Store Write1 : DataStoreWrite  DataStoreName=RefTmrLrngConstr
  Data Store Write2 : DataStoreWrite  DataStoreName=RefTmrNtc
  FricChgLpFil : Fil/FilLpInit  Ic=0  Ts=ARCHGLBPRM_10MILLISEC_SEC_F32  Freq=SysFricLrngFricOffsLpFilFrq  StVar=FricChgLpFil
  GetRefTmr100MicroSec32bit : Subsystem
  GetRefTmr100MicroSec32bit1 : Subsystem
  HwAgAuthyLpFil : Fil/FilLpInit  Ic=0  Ts=ARCHGLBPRM_10MILLISEC_SEC_F32  Freq=SysFricLrngDataPrepLpFilFrq  StVar=HwAgAuthyLpFil
  HwAgLpFil : Fil/FilLpInit  Ic=0  Ts=ARCHGLBPRM_10MILLISEC_SEC_F32  Freq=SysFricLrngDataPrepLpFilFrq  StVar=HwAgLpFil
  HwVelLpFil : Fil/FilLpInit  Ic=0  Ts=ARCHGLBPRM_10MILLISEC_SEC_F32  Freq=SysFricLrngDataPrepLpFilFrq  StVar=HwVelLpFil
  Initialization : Subsystem  RequirementInfo={} %GIDa_91d738c7_e712_4f5c_81ea_e86a6bba312a  Priority=1  TreatAsAtomicUnit=on
  LatALpFil : Fil/FilLpInit  Ic=0  Ts=ARCHGLBPRM_10MILLISEC_SEC_F32  Freq=SysFricLrngDataPrepLpFilFrq  StVar=LatALpFil
  Set Ram Block Status : NxtrNvM/Set Ram Block Status  FuncName=Set Ram Block Status  NvMBlockName=FricLrngData  VoidFuncRtn=on  BlockChanged_DSN=NvMSRBS_BlockChanged  Return_DSN=NvMSRBS_Return
      settings: AttributesFormatString=%<FuncName>
  VehSpdLpFil : Fil/FilLpInit  Ic=0  Ts=ARCHGLBPRM_10MILLISEC_SEC_F32  Freq=SysFricLrngDataPrepLpFilFrq  StVar=VehSpdLpFil
  SysFricOffs : Outport
  wires:
  Data Store Read/1 -> Data Store Write/1
  GetRefTmr100MicroSec32bit/1(RefTmr) -> Data Store Write1/1
  Constant/1 -> Initialization/1(VEHSPDPTNUM1_ULS_U08)
  Data Store Read1/1 -> SysFricOffs/1
  GetRefTmr100MicroSec32bit1/1(RefTmr) -> Data Store Write2/1
  Constant1/1 -> Set Ram Block Status/1

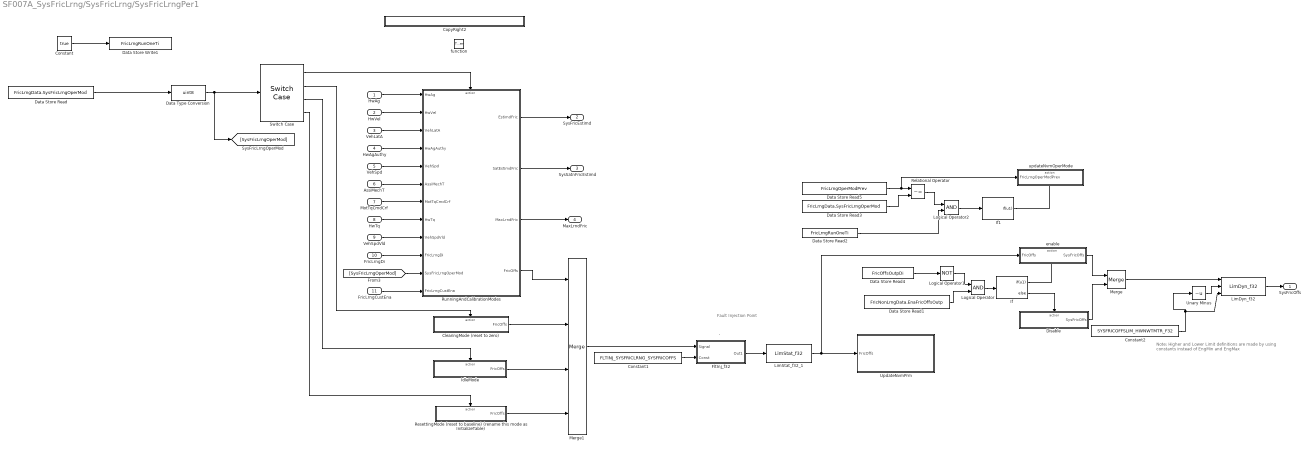
== system SF007A_SysFricLrng/SysFricLrng/SysFricLrngPer1 ==
  note: ,
  note: Fault
      | Injection
      | Point
  note: Note: Higher and Lower Limit definitions are made
      |           by using constants instead of EngMin and EngMax
  HwAg : Inport
  HwVel : Inport  Port=2
  VehLatA : Inport  Port=3
  HwAgAuthy : Inport  Port=4
  VehSpd : Inport  Port=5
  AssiMechT : Inport  Port=6
  MotTqCmdCrf : Inport  Port=7
  HwTq : Inport  Port=8
  VehSpdVld : Inport  Port=9
  FricLrngDi : Inport  Port=10
  FricLrngCustEna : Inport  Port=11
  function : TriggerPort  TriggerType=function-call
  ClearingMode (reset to zero) : Subsystem
  Constant : Constant  Value=true  OutDataTypeStr=boolean
      settings: AttributesFormatString=%<OutDataTypeStr>
  Constant1 : Constant  Value=FLTINJ_SYSFRICLRNG_SYSFRICOFFS  SampleTime=-1
  Constant2 : Constant  Value=SYSFRICOFFSLIM_HWNWTMTR_F32  SampleTime=-1
  CopyRight2 : Subsystem  Description=|  mask(Copyright Information){none=on}
      | Copyright info block.                                               
      |                                                                     
      | Place copyright information at the top of every subsystem in design.
      mask prompts: none "No parameters"
      mask help: Place copyright information at the top of every subsystem in design.
      mask Display:
      | NxtrConf = 'Nexteer Confidential';
      | 
      | sys = bdroot; %handle for the current model ("system")
      | first = get_param(sys,'Created');
      | if(isempty(first))
      |     first = datestr(now,'yyyy');
      | else
      |     first = first(end-3:end);  %year is last four digits
      | end
      | 
      | last = get_param(sys,'LastModifiedDate');
      | if isempty(last)
      |     last = datestr(now,'yyyy');
      | else
      |     last = last(end-3:end);
      | end
      | 
      | if strcmp(first,last)
      |     fprintf('%s -- Copyright %s Nexteer',NxtrConf,first)
      | else
      |     fprintf('%s -- %s%s- %s Nexteer',NxtrConf,char(169),first,last)
      | end
  Data Store Read : DataStoreRead  DataStoreName=FricLrngData  DataStoreElements=FricLrngData.SysFricLrngOperMod
  Data Store Read1 : DataStoreRead  DataStoreName=FricNonLrngData  DataStoreElements=FricNonLrngData.EnaFricOffsOutp
  Data Store Read2 : DataStoreRead  DataStoreName=FricLrngRunOneTi
  Data Store Read3 : DataStoreRead  DataStoreName=FricLrngData  DataStoreElements=FricLrngData.SysFricLrngOperMod
  Data Store Read4 : DataStoreRead  DataStoreName=FricOffsOutpDi
  Data Store Read5 : DataStoreRead  DataStoreName=FricLrngOperModPrev
  Data Store Write1 : DataStoreWrite  DataStoreName=FricLrngRunOneTi
  Data Type Conversion : DataTypeConversion  OutDataTypeStr=uint8
  Disable : Subsystem  TreatAsAtomicUnit=on
  FltInj_f32 : Subsystem  RequirementInfo={} %GIDa_0b9e84c1_4f47_4480_b4c5_5d0515f10b4a  TreatAsAtomicUnit=on  VariantControl=FltInj_sim  mask(Fault_Injection){}
      mask help: Fault Injection is a simulation only block for EA4 programs.
  IdleMode : Subsystem
  If : If  IfExpression=u1
  If1 : If  IfExpression=u1  ShowElse=off
  LimDyn_f32 : NxtrLim/LimDyn_f32
  LimStat_f32_1 : NxtrLim/LimStat_f32  LoLim=SysFricLrngFricOffsLoLim  HiLim=SysFricLrngFricOffsHiLim
      settings: AttributesFormatString=|
      | Low Limit: %<LoLim>
      | High Limit:%<HiLim>
  Logical Operator : Logic  AllPortsSameDT=off  OutDataTypeStr=boolean
  Logical Operator1 : Logic  Operator=NOT  AllPortsSameDT=off  OutDataTypeStr=boolean
  Logical Operator2 : Logic  AllPortsSameDT=off  OutDataTypeStr=boolean
  Merge : Merge
  Merge1 : Merge  Inputs=4
  Relational Operator : RelationalOperator  Operator=~=  OutDataTypeStr=boolean
  ResettingMode (reset to baseline) (rename this mode as InitializeTable) : Subsystem
  RunningAndCalibrationModes : Subsystem
  Switch Case : SwitchCase  CaseConditions={[0,1],2,3}
  Unary Minus : UnaryMinus
  UpdateNvmPrm : Subsystem
  enable : Subsystem  TreatAsAtomicUnit=on
  updateNvmOperMode : Subsystem  TreatAsAtomicUnit=on
  SysFricOffs : Outport
  SysFricEstimd : Outport  Port=2
  SysSatnFricEstimd : Outport  Port=3
  MaxLrndFric : Outport  Port=4
  wires:
  HwAg/1 -> RunningAndCalibrationModes/1(HwAg)
  HwVel/1 -> RunningAndCalibrationModes/2(HwVel)
  VehLatA/1 -> RunningAndCalibrationModes/3(VehLatA)
  HwAgAuthy/1 -> RunningAndCalibrationModes/4(HwAgAuthy)
  VehSpd/1 -> RunningAndCalibrationModes/5(VehSpd)
  AssiMechT/1 -> RunningAndCalibrationModes/6(AssiMechT)
  MotTqCmdCrf/1 -> RunningAndCalibrationModes/7(MotTqCmdCrf)
  HwTq/1 -> RunningAndCalibrationModes/8(HwTq)
  [SysFricLrngOperMod] -> RunningAndCalibrationModes/11(SysFricLrngOperMod)
  VehSpdVld/1 -> RunningAndCalibrationModes/9(VehSpdVld)
  Merge/1 -> LimDyn_f32/1
  Logical Operator1/1 -> Logical Operator/1
  Logical Operator/1 -> If/1
  LimStat_f32_1/1 -> enable/1(FricOffs), UpdateNvmPrm/1(FricOffs)
  Data Store Read1/1 -> Logical Operator/2
  FricLrngDi/1 -> RunningAndCalibrationModes/10(FricLrngDi)
  If/1 -> enable/Action
  If/2 -> Disable/Action
  enable/1("SysFricOffs ") -> Merge/1
  Disable/1(SysFricOffs) -> Merge/2
  Data Store Read/1 -> Data Type Conversion/1
  Switch Case/1 -> RunningAndCalibrationModes/Action
  Switch Case/2 -> ClearingMode (reset to zero)/Action
  Switch Case/3 -> IdleMode/Action
  Switch Case/4 -> ResettingMode (reset to baseline) (rename this mode as InitializeTable)/Action
  RunningAndCalibrationModes/4(FricOffs) -> Merge1/1
  ClearingMode (reset to zero)/1(FricOffs) -> Merge1/2
  IdleMode/1(FricOffs) -> Merge1/3
  ResettingMode (reset to baseline) (rename this mode as InitializeTable)/1(FricOffs) -> Merge1/4
  Data Type Conversion/1 -> Switch Case/1, [SysFricLrngOperMod]
  Merge1/1 -> FltInj_f32/1(Signal)
  FltInj_f32/1(Out1) -> LimStat_f32_1/1
  Constant1/1 -> FltInj_f32/2(Const)
  RunningAndCalibrationModes/2(SatEstimdFric) -> SysSatnFricEstimd/1
  RunningAndCalibrationModes/1(EstimdFric) -> SysFricEstimd/1
  FricLrngCustEna/1 -> RunningAndCalibrationModes/12(FricLrngCustEna)
  Data Store Read4/1 -> Logical Operator1/1
  Constant/1 -> Data Store Write1/1
  Relational Operator/1 -> Logical Operator2/1
  Data Store Read2/1 -> Logical Operator2/2
  Data Store Read5/1 -> updateNvmOperMode/1(FricLrngOperModPrev), Relational Operator/1
  Data Store Read3/1 -> Relational Operator/2
  Logical Operator2/1 -> If1/1
  If1/1 -> updateNvmOperMode/Action
  RunningAndCalibrationModes/3(MaxLrndFric) -> MaxLrndFric/1
  LimDyn_f32/1 -> SysFricOffs/1
  Unary Minus/1 -> LimDyn_f32/2
  Constant2/1 -> LimDyn_f32/3, Unary Minus/1

== system SF007A_SysFricLrng/call_SysFricLrngInit1/CopyRight2 ==

== system SF007A_SysFricLrng/call_SysFricLrngPer1/CopyRight2 ==

== system SF007A_SysFricLrng/SysFricLrng/ClrFricLrngOperMod/CopyRight2 ==

== system SF007A_SysFricLrng/SysFricLrng/GetFricLrngData/CopyRight2 ==

== system SF007A_SysFricLrng/SysFricLrng/GetFricOffsOutpDi/CopyRight2 ==
